simulink model "current_control_2015"  (R2020a)
settings: Solver=ode4  StartTime=0.0  StopTime=inf  FixedStep=0.001  RelTol=1e-3  EnableMultiTasking=on
undefined symbols (not defined in the file): gains_increasing, Kp_i_increasing, L, Ti_i_increasing, x, x_eq_increasing, y
libraries: PoliArd x7
settings Model: ExtModeTrigDuration=2  Creator=User  LastModifiedBy=miche
settings DataIOCC: LimitDataPoints=on  SaveFormat=Array  ReturnWorkspaceOutputs=off
settings OptimizationCC: LifeSpan=1  EfficientTunableParamExpr=on
settings DebuggingCC: UnderspecifiedInitializationDetection=Classic  MergeDetectMultiDrivingBlocksExec=none  SFUnexpectedBacktrackingDiag=warning  SFNoUnconditionalDefaultTransitionDiag=warning  SFExecutionAtInitializationDiag=none  ArithmeticOperatorsInVariantConditions=warning
settings HardwareCC: ProdBitPerPointer=32  ProdBitPerSizeT=32  ProdBitPerPtrDiffT=32  ProdLargestAtomicInteger=Long  ProdLargestAtomicFloat=Double  ProdIntDivRoundTo=Undefined  ProdWordSize=32  ProdHWDeviceType=ARM Compatible->ARM Cortex
settings ModelReferenceCC: PropagateSignalLabelsOutOfModel=off
settings SFSimCC: SimUseLocalCustomCode=off  MATLABDynamicMemAlloc=off  CustomCodeUndefinedFunction=UseInterfaceOnly
settings RTWCC: Description=Run on Target Hardware  SystemTargetFile=realtime.tlc  GenerateMakefile=off  TemplateMakefile=realtime.tmf  RTWVerbose=off  RTWUseLocalCustomCode=off
settings CodeAppCC: StateflowObjectComments=on
settings STFCustomTargetCC: TargetLibSuffix=.a  GenerateSampleERTMain=on  ERTCustomFileBanners=on  SupportNonInlinedSFcns=off  RemoveResetFunc=on  SupportVariableSizeSignals=on  MATLABClassNameForMDSCustomization=Simulink.SoftwareTarget.ERTCustomization  SystemTargetFile=realtime.tlc
settings ERTTargetCC: MultiwordLength=2048  GenerateSampleERTMain=on  ParMdlRefBuildCompliant=off  CompOptLevelCompliant=off  ConcurrentExecutionCompliant=off  CombineOutputUpdateFcns=off  SupportContinuousTime=on  SupportVariableSizeSignals=on  ModelStepFunctionPrototypeControlCompliant=off  CPPClassGenCompliant=off  UseToolchainInfoCompliant=off  ExtModeTransport=3  ExtModeMexFile=ext_serial_win32_comm_rtt  ExtModeMexArgs=0 1 9600  ERTSrcFileBannerTemplate=realtime_code_template.cgt  ERTHdrFileBannerTemplate=realtime_code_template.cgt  ERTDataSrcFileTemplate=realtime_code_template.cgt  ERTDataHdrFileTemplate=realtime_code_template.cgt  ERTCustomFileTemplate=realtime_file_process.tlc  ConvertIfToSwitch=off  SuppressUnreachableDefaultCases=off
settings ConfigComp: CovMetricSettings=dw  CovSaveCumulativeToWorkspaceVar=on  CovSaveSingleToWorkspaceVar=on  CovExternalEMLEnable=off

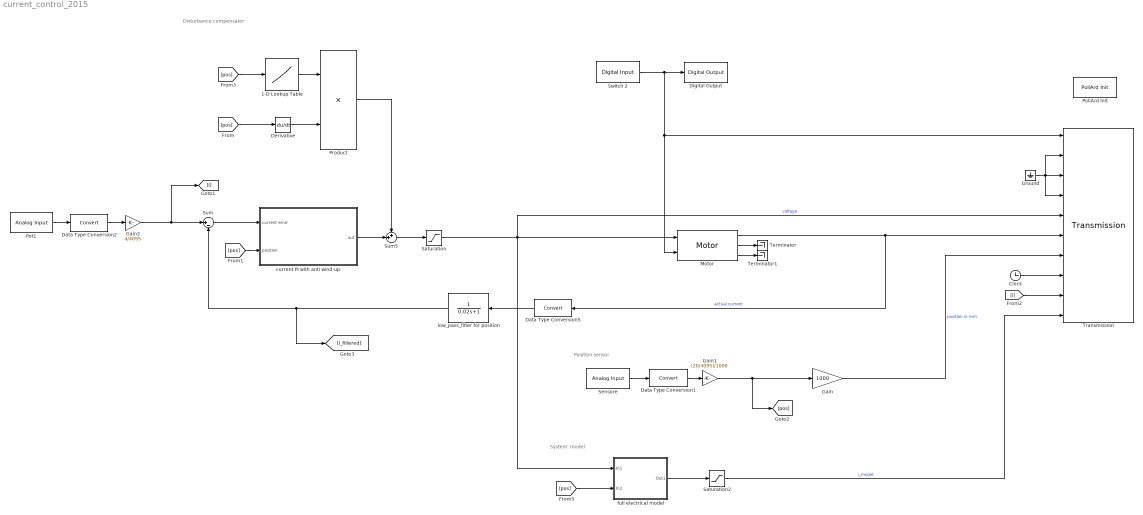
== system current_control_2015 ==
  note: System' model
  note: Position sensor
  note: Disturbance compensator
  1-D Lookup Table : Lookup_n-D  NumberOfTableDimensions=1  BreakpointsForDimension1=[0.0085 x_eq_increasing]  Table=[gains_increasing(1) gains_increasing]  InternalRulePriority=Speed  RndMeth=Simplest  InputSameDT=on
  Clock : Clock
  Data Type Conversion1 : DataTypeConversion
  Data Type Conversion2 : DataTypeConversion
  Data Type Conversion5 : DataTypeConversion
  Derivative : Derivative
  Digital Output : PoliArd/Digital Output  DO_pin=1
  Gain : Gain  Gain=1000
  Gain1 : Gain  Gain=(20/4095)/1000
  Gain2 : Gain  Gain=4/4095
  Ground : Ground
  Motor : PoliArd/Motor  MotorID=2  DC_bus_mask=24  dt_mot=-1
  PoliArd Init : PoliArd/PoliArd Init
  Pot1 : PoliArd/Analog Input  AIpin_mask=8  AIsample=-1
  Product : Product
  Saturation : Saturate  UpperLimit=16  LowerLimit=0
  Saturation2 : Saturate  UpperLimit=4  LowerLimit=0
  Sensore : PoliArd/Analog Input  AIpin_mask=2  AIsample=-1
  Sum : Sum  Inputs=|+-
  Sum5 : Sum  Inputs=++|
  Switch 2 : PoliArd/Digital Input  DI_pin=2  DIsample=-1
  Terminator : Terminator
  Terminator1 : Terminator
  Transmission : PoliArd/Transmission  sample_freq=1000  sig_to_send=6
  current PI with anti wind-up : Subsystem
      mask Display: disp('Current controller\n(PI)\nwith anti wind-up')
  full electrical model : Subsystem
      mask Display: disp('Full electrical\nmodel')
  low_pass_filter for position : TransferFcn  Denominator=[0.02 1]
  wires:
  [pos] -> Derivative/1
  Derivative/1 -> Product/2
  Sum/1 -> current PI with anti wind-up/1(current error)
  Sum5/1 -> Saturation/1
  Product/1 -> Sum5/1
  Saturation/1 -> Motor/1, Transmission/5, full electrical model/1(In1)  "voltage"
  Data Type Conversion2/1 -> Gain2/1
  Data Type Conversion5/1 -> low_pass_filter for position/1
  [pos] -> 1-D Lookup Table/1
  1-D Lookup Table/1 -> Product/1
  Gain1/1 -> [pos], Gain/1
  Data Type Conversion1/1 -> Gain1/1
  Switch 2/1 -> Digital Output/1, Motor/2, Transmission/1
  Ground/1 -> Transmission/2, Transmission/4, Transmission/3
  Motor/1 -> Transmission/6, Data Type Conversion5/1  "actual current"
  Sensore/1 -> Data Type Conversion1/1
  [i] -> Transmission/9
  Clock/1 -> Transmission/8
  low_pass_filter for position/1 -> Sum/2, [i_filtered]
  Gain/1 -> Transmission/7  "position in mm"
  current PI with anti wind-up/1(out) -> Sum5/2
  [pos] -> current PI with anti wind-up/2(position)
  Motor/2 -> Terminator/1
  Motor/3 -> Terminator1/1
  full electrical model/1(Out1) -> Saturation2/1
  [pos] -> full electrical model/2(In2)
  Saturation2/1 -> Transmission/10  "i_model"
  Pot1/1 -> Data Type Conversion2/1
  Gain2/1 -> Sum/1, [i]

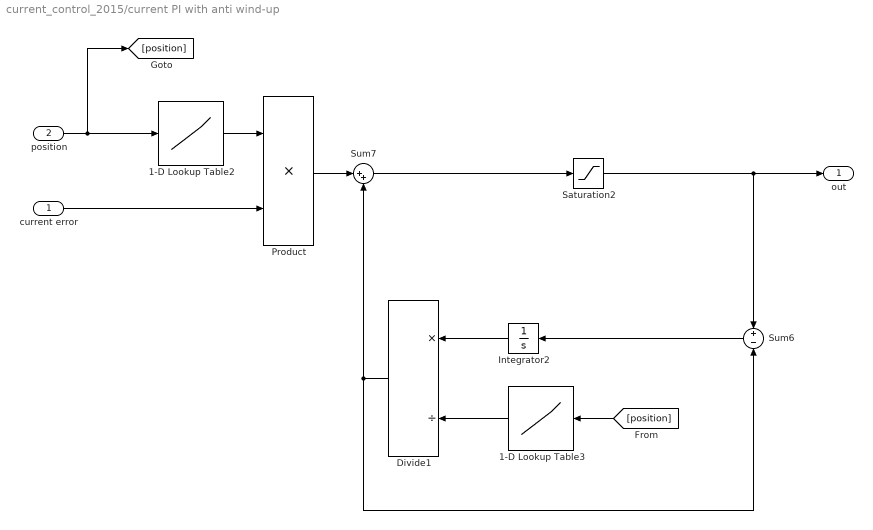
== system current_control_2015/current PI with anti wind-up ==
  current error : Inport
  position : Inport  Port=2
  1-D Lookup Table2 : Lookup_n-D  NumberOfTableDimensions=1  BreakpointsForDimension1=[0.0085 x_eq_increasing]  Table=[Kp_i_increasing(1) Kp_i_increasing]  InternalRulePriority=Speed  RndMeth=Simplest  InputSameDT=on
  1-D Lookup Table3 : Lookup_n-D  NumberOfTableDimensions=1  BreakpointsForDimension1=[0.0085 x_eq_increasing]  Table=[Ti_i_increasing(1) Ti_i_increasing]  InternalRulePriority=Speed  RndMeth=Simplest  InputSameDT=on
  Divide1 : Product  Inputs=*/
  Integrator2 : Integrator
  Product : Product
  Saturation2 : Saturate  UpperLimit=16  LowerLimit=0
  Sum6 : Sum  Inputs=+|-
  Sum7 : Sum  Inputs=|++
  out : Outport
  wires:
  Sum7/1 -> Saturation2/1
  Product/1 -> Sum7/1
  Saturation2/1 -> out/1, Sum6/1
  current error/1 -> Product/2
  1-D Lookup Table2/1 -> Product/1
  position/1 -> [position], 1-D Lookup Table2/1
  Divide1/1 -> Sum6/2, Sum7/2
  Sum6/1 -> Integrator2/1
  Integrator2/1 -> Divide1/1
  1-D Lookup Table3/1 -> Divide1/2
  [position] -> 1-D Lookup Table3/1

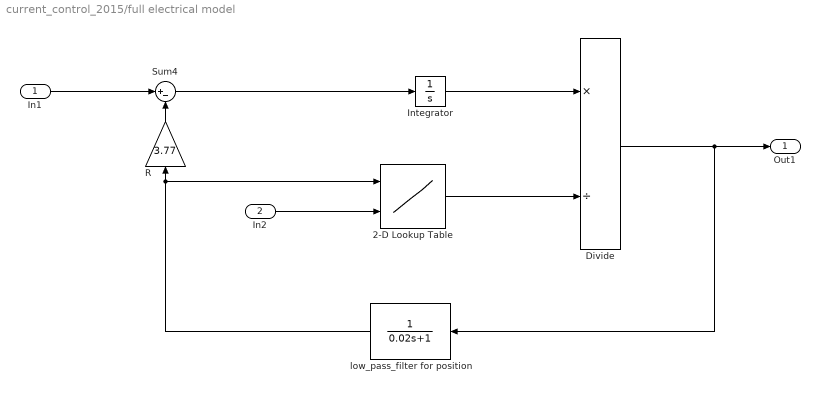
== system current_control_2015/full electrical model ==
  In1 : Inport
  In2 : Inport  Port=2
  2-D Lookup Table : Lookup_n-D  BreakpointsForDimension1=y  BreakpointsForDimension2=x  Table=L  InternalRulePriority=Speed  RndMeth=Simplest  InputSameDT=on
  Divide : Product  Inputs=*/
  Integrator : Integrator
  R : Gain  Gain=3.77
  Sum4 : Sum  Inputs=|+-
  low_pass_filter for position : TransferFcn  Denominator=[0.02 1]
  Out1 : Outport
  wires:
  Sum4/1 -> Integrator/1
  Integrator/1 -> Divide/1
  R/1 -> Sum4/2
  In2/1 -> 2-D Lookup Table/2
  2-D Lookup Table/1 -> Divide/2
  In1/1 -> Sum4/1
  Divide/1 -> Out1/1, low_pass_filter for position/1
  low_pass_filter for position/1 -> R/1, 2-D Lookup Table/1
